simulink model "scdmultiplechecks"  (Simulink 7.6)
settings: Solver=ode45  StartTime=0.0  StopTime=Tend  MaxStep=15*60  RelTol=1e-3
model workspace (MATLAB code in the model file):
  | %Fixed values. Based on typical long-haul commerical aircraft
  | mFuel  = 160000;   %kg
  | mTotal = 300000;   %kg
  | vCruise =240;  %m/s
  | A = 1000;  %m^2
  | Cd = 0.031;   %Draft coeff
  | rhoAir = 1.4/4;  %kg/m^3
  | Kengine = 65400;  %kg*m/s^2
  | Tend   = 60*60*8;
  | 
  | %Derived values
  | kv0 = 0.75;
  | mVehicle = mTotal-mFuel;
  | cDrag = 0.5*rhoAir*Cd*A;
  | c0 = (kv0*vCruise)^2*cDrag/Kengine;
undefined symbols (not defined in the file or in its folder): magnitude, sigbuilder_block
libraries: simulink x2, slctrlblks x1
settings Model: Creator=The MathWorks Inc.  BufferReuse=off
settings OptimizationCC: BlockReduction=off  InlineParams=on  BufferReuse=off

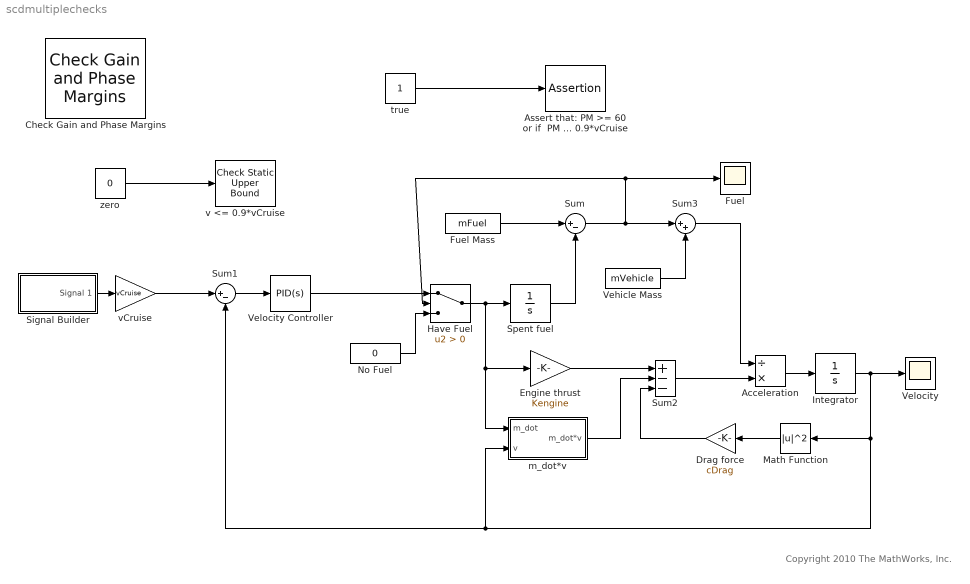
== system scdmultiplechecks ==
  note: Copyright 2010 The MathWorks, Inc.
  Acceleration : Product  Inputs=/*  SaturateOnIntegerOverflow=on  RndMeth=Zero  InputSameDT=on  OutDataTypeStr=Inherit: Same as first input
  Assert that: PM >= 60 or if  PM < 60 then v <= 0.9*vCruise : Assertion  Enabled=on
  Check Gain and Phase Margins : slctrlblks/Model Verification/Check Gain and Phase Margins  InstantiateOnLoad=on  DialogController=checkpack.createCheckDlg  DialogControllerArgs=DataTag0  SystemSampleTime=-1  LinearizationIOs={'/Velocity Controller ', 1, 'outin', 'on'}  LinearizeAt=SnapshotTimes  SnapshotTimes=0:30*60:Tend  TriggerType=rising  ZeroCross=off  SampleTime=auto  RateConversionMethod=zoh  PreWarpFreq=10  UseExactDelayModel=off  UseFullBlockNameLabels=off  UseBusSignalLabels=off  enabled=on  stopWhenAssertionFail=off  export=off  ViewDlgPos=[67 135 510 631]  LaunchViewOnOpen=off  OpenViewOnLoad=off  FrequencyUnits=rad/sec  MagnitudeUnits=dB  PhaseUnits=deg  EnableMargins=on  GainMargin=20  PhaseMargin=30  PlotType=bode  FeedbackSign=-1
      settings: SaveToWorkspace=on  SaveName=LinearAircraft
  Drag force : Gain  Gain=cDrag  SaturateOnIntegerOverflow=on  OutDataTypeStr=Inherit: Same as input  ParamDataTypeStr=Inherit: Same as input
  Engine thrust : Gain  Gain=Kengine  SaturateOnIntegerOverflow=on  OutDataTypeStr=Inherit: Same as input  ParamDataTypeStr=Inherit: Same as input
  Fuel : Scope
      settings: TimeRange=30000  YMin=0  YMax=200000
  Fuel Mass : Constant  Value=mFuel
  Have Fuel : Switch  Criteria=u2 > Threshold
  Integrator : Integrator  InitialCondition=kv0*vCruise  LimitOutput=on  LowerSaturationLimit=0
  Math Function : Math  Operator=magnitude^2  SaturateOnIntegerOverflow=on
  No Fuel : Constant  Value=0
  Signal Builder : Subsystem  Tag=STV Subsys  LoadFcn=sigbuilder_block('load');  StartFcn=sigbuilder_block('start');  StopFcn=sigbuilder_block('stop');  ClipboardFcn=sigbuilder_block('clipboard');  mask(Sigbuilder block){}
      mask help: Create and generate interchangeable groups of signals whose waveforms are piecewise linear.
      mask init:
      | if ~strcmp(get_param(bdroot(gcbh),'SimulationStatus'),'stopped') tuvar = sigbuilder_block('maskInit'); end
      settings: CopyFcn=sigbuilder_block('copy');  DeleteFcn=sigbuilder_block('delete');  ModelCloseFcn=sigbuilder_block('modelClose');  PreSaveFcn=sigbuilder_block('preSave');  NameChangeFcn=sigbuilder_block('namechange');  OpenFcn=sigbuilder_block('open',[840.75 369.75 550.5 399.75 ]);  CloseFcn=sigbuilder_block('close');
      mask Display: plot(0,0,100,100,[10,10,40,40,10],[80,20,20,80,80],[40,10],[50,50], [40,27,10],[65,72,56],[40,25,25,10],[28,28,43,43]);
  Spent fuel : Integrator  SCDEnableBlockLinearizationSpecification=on  LowerSaturationLimit=0
  Sum : Sum  Inputs=|+-
  Sum1 : Sum  Inputs=|+-
  Sum2 : Sum  Inputs=+--
  Sum3 : Sum  Inputs=|++
  Vehicle Mass : Constant  Value=mVehicle
  Velocity : Scope
      settings: TimeRange=30000  YMin=180  YMax=300  SaveName=ScopeData2
  "Velocity Controller " : simulink/Continuous/PID Controller  DialogController=pidpack.PIDConfig.pidDDGCreate  DialogControllerArgs=DataTag3  SystemSampleTime=-1  Controller=PID  TimeDomain=Continuous-time  SampleTime=1  IntegratorMethod=Forward Euler  FilterMethod=Forward Euler  Form=Parallel  P=0.749203308944003  I=0.0118377140035095  D=-1.73193766119674  N=0.403766652570375  InitialConditionSource=internal  InitialConditionForIntegrator=c0  InitialConditionForFilter=0  ExternalReset=none  LimitOutput=on  UpperSaturationLimit=inf  LowerSaturationLimit=0  LinearizeAsGain=off  AntiWindupMode=clamping  Kb=1  TrackingMode=off  Kt=1  PParamMin=[]  PParamMax=[]  IParamMin=[]  IParamMax=[]  DParamMin=[]  DParamMax=[]  NParamMin=[]  NParamMax=[]  KbParamMin=[]  KbParamMax=[]  KtParamMin=[]  KtParamMax=[]  POutMin=[]  POutMax=[]  IOutMin=[]  IOutMax=[]  DOutMin=[]  DOutMax=[]  NOutMin=[]  NOutMax=[]  KbOutMin=[]  KbOutMax=[]  KtOutMin=[]  KtOutMax=[]  IntegratorOutMin=[]  IntegratorOutMax=[]  FilterOutMin=[]  FilterOutMax=[]  SumOutMin=[]  SumOutMax=[]  SumI1OutMin=[]  SumI1OutMax=[]  SumI2OutMin=[]  SumI2OutMax=[]  SumI3OutMin=[]  SumI3OutMax=[]  SumDOutMin=[]  SumDOutMax=[]  SaturationOutMin=[]  SaturationOutMax=[]  IntegratorContinuousStateAttributes=''  IntegratorStateMustResolveToSignalObject=off  IntegratorRTWStateStorageClass=Auto  FilterContinuousStateAttributes=''  FilterStateMustResolveToSignalObject=off  FilterRTWStateStorageClass=Auto
  m_dot*v : Subsystem
  true : Constant
  v <= 0.9*vCruise : simulink/Model Verification/Check Static  Upper Bound  Description=u <= 0  SystemSampleTime=-1  max=0  max_included=on  enabled=on  stopWhenAssertionFail=on  export=off  icon=graphic
  vCruise : Gain  Gain=vCruise  SaturateOnIntegerOverflow=on  OutDataTypeStr=Inherit: Same as input  ParamDataTypeStr=Inherit: Same as input
  zero : Constant  Value=0
  wires:
  Integrator/1 -> Math Function/1, Sum1/2, m_dot*v/2(v), Velocity/1
  No Fuel/1 -> Have Fuel/3
  Sum1/1 -> "Velocity Controller "/1
  Spent fuel/1 -> Sum/2
  Sum/1 -> Sum3/1, Have Fuel/2, Fuel/1
  Acceleration/1 -> Integrator/1
  Sum2/1 -> Acceleration/2
  Engine thrust/1 -> Sum2/1
  Drag force/1 -> Sum2/3
  Have Fuel/1 -> Spent fuel/1, Engine thrust/1, m_dot*v/1(m_dot)
  "Velocity Controller "/1 -> Have Fuel/1
  Fuel Mass/1 -> Sum/1
  Sum3/1 -> Acceleration/1
  Vehicle Mass/1 -> Sum3/2
  Math Function/1 -> Drag force/1
  vCruise/1 -> Sum1/1
  Signal Builder/1(Signal 1) -> vCruise/1
  true/1 -> Assert that: PM >= 60 or if  PM < 60 then v <= 0.9*vCruise/1
  zero/1 -> v <= 0.9*vCruise/1
  m_dot*v/1(m_dot*v) -> Sum2/2

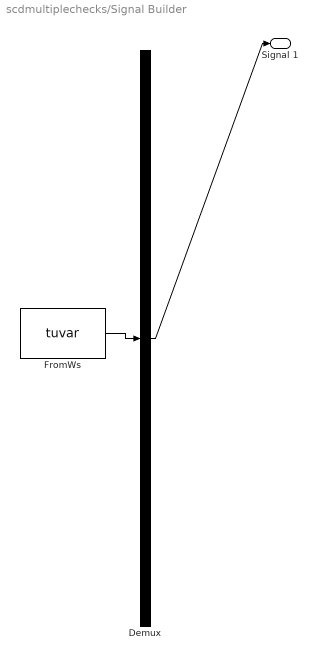
== system scdmultiplechecks/Signal Builder ==
  Demux : Demux  Tag=STV Demux  Outputs=1
  FromWs : FromWorkspace  Tag=STV FromWs  VariableName=tuvar  SampleTime=0  SigBuilderData=DataTag1  VnvData=DataTag2
      SigBuilderData=|
      | common.afterFinalStr = 'Extrapolate'
      | common.sampleTime = 0
      | dataSet.timeRange = [0 28800]
      | dataSet.name = 'Group 1'
      | sbobj.Groups.Name = 'Group 1'
      | sbobj.Groups.Signals.Name = 'Signal 1'
      | sbobj.Groups.Signals.XData = [0 3600 7000 8800 12000 13800 13800 20000 28800]
      | sbobj.Groups.Signals.YData = [0.752 1 1 1.05 1.05 1 1.002 1 0.75]
      | sbobj.Groups.TimeRange = [0 28800]
  Signal 1 : Outport  Tag=STV Outport
  wires:
  FromWs/1 -> Demux/1
  Demux/1 -> Signal 1/1

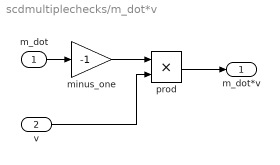
== system scdmultiplechecks/m_dot*v ==
  m_dot : Inport
  v : Inport  Port=2
  minus_one : Gain  Gain=-1  SaturateOnIntegerOverflow=on  OutDataTypeStr=Inherit: Same as input  ParamDataTypeStr=Inherit: Same as input
  prod : Product  Inputs=**  SaturateOnIntegerOverflow=on  RndMeth=Zero  InputSameDT=on  OutDataTypeStr=Inherit: Same as first input
  m_dot*v : Outport
  wires:
  prod/1 -> m_dot*v/1
  v/1 -> prod/2
  m_dot/1 -> minus_one/1
  minus_one/1 -> prod/1
